simulink model "my_model"  (R2025a)
settings: Solver=FixedStepAuto  StartTime=0.0  StopTime=10.0  RelTol=1e-3
values from neighbouring files (symbols this model uses):
  net = block.UserData    [NN_MPC_SFunction.m]
undefined symbols (not defined in the file or in its folder): getString, message
libraries: dlconvfclib x3, dlactivationlib x2
settings Model: Creator=thapl  LastModifiedBy=thapl
settings OptimizationCC: DefaultParameterBehavior=Inlined  EnhancedBackFolding=on  PassReuseOutputArgsAs=Individual arguments  ZeroExternalMemoryAtStartup=off  ZeroInternalMemoryAtStartup=off  OptimizeBlockOrder=speed  DifferentSizesBufferReuse=on  OptimizationCustomize=off  EfficientTunableParamExpr=on
settings DebuggingCC: ParameterTunabilityLossMsg=error
settings SFSimCC: MATLABDynamicMemAlloc=off
settings RTWCC: SystemTargetFile=ert.tlc  TemplateMakefile=ert_default_tmf  Description=Embedded Coder
settings CodeAppCC: ForceParamTrailComments=on  IgnoreCustomStorageClasses=off  OperatorAnnotations=on  SimulinkDataObjDesc=on  SFDataObjDesc=on  InsertBlockDesc=on
settings ERTTargetCC: ExtModeTransport=0.0  ExtModeStaticAlloc=off  ExtModeMexFile=ext_comm  ExtModeIntrfLevel=Level1  ERTCustomFileTemplate=example_file_process.tlc  TargetLangStandard=C99 (ISO)  GenerateSampleERTMain=on

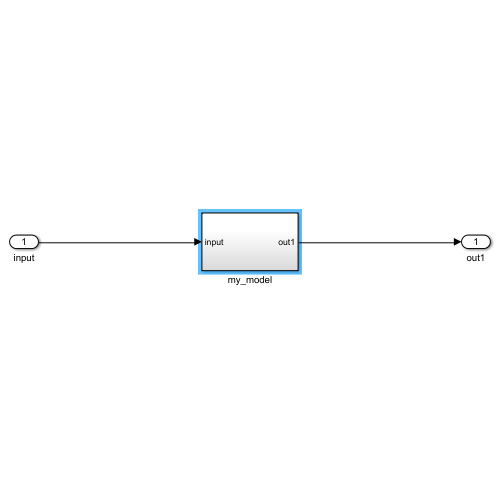
[thumbnail: Simulink's stored preview of the top-level diagram]
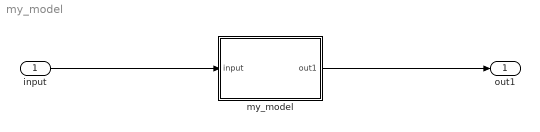
== system my_model ==
  input : Inport  PortDimensions=[20]
  my_model : Subsystem
  out1 : Outport
  wires:
  input/1 -> my_model/1(input)
  my_model/1(out1) -> out1/1

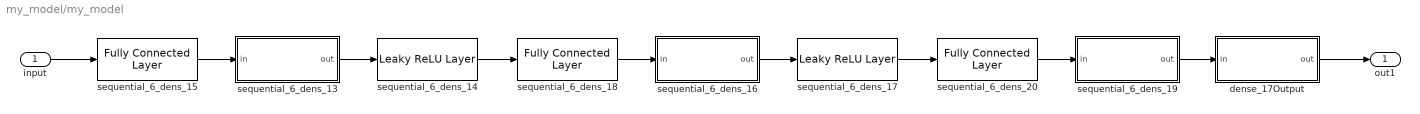
== system my_model/my_model ==
  input : Inport  PortDimensions=[20]
  dense_17Output : Subsystem
  sequential_6_dens_13 : Subsystem
  sequential_6_dens_14 : dlactivationlib/Leaky ReLU Layer  Scale=net.Layers(4).Scale  OutMin=[]  OutMax=[]  ScaleDataTypeStr=Inherit: Inherit via back propagation  ScaleMin=[]  ScaleMax=[]  InternalRndMeth=Floor  InternalSaturateOnIntegerOverflow=off  SampleTime=-1
  sequential_6_dens_15 : dlconvfclib/Fully Connected Layer  Layer=net.Layers(2)  OutMin=[]  OutMax=[]  WeightsDataTypeStr=Inherit: Inherit via back propagation  WeightsMin=[]  WeightsMax=[]  BiasDataTypeStr=Inherit: Inherit via back propagation  BiasMin=[]  BiasMax=[]  AccumMin=[]  AccumMax=[]  InternalRndMeth=Floor  InternalSaturateOnIntegerOverflow=off  SampleTime=-1
      settings: DataFormat=C
  sequential_6_dens_16 : Subsystem
  sequential_6_dens_17 : dlactivationlib/Leaky ReLU Layer  Scale=net.Layers(7).Scale  OutMin=[]  OutMax=[]  ScaleDataTypeStr=Inherit: Inherit via back propagation  ScaleMin=[]  ScaleMax=[]  InternalRndMeth=Floor  InternalSaturateOnIntegerOverflow=off  SampleTime=-1
  sequential_6_dens_18 : dlconvfclib/Fully Connected Layer  Layer=net.Layers(5)  OutMin=[]  OutMax=[]  WeightsDataTypeStr=Inherit: Inherit via back propagation  WeightsMin=[]  WeightsMax=[]  BiasDataTypeStr=Inherit: Inherit via back propagation  BiasMin=[]  BiasMax=[]  AccumMin=[]  AccumMax=[]  InternalRndMeth=Floor  InternalSaturateOnIntegerOverflow=off  SampleTime=-1
      settings: DataFormat=C
  sequential_6_dens_19 : Subsystem
  sequential_6_dens_20 : dlconvfclib/Fully Connected Layer  Layer=net.Layers(8)  OutMin=[]  OutMax=[]  WeightsDataTypeStr=Inherit: Inherit via back propagation  WeightsMin=[]  WeightsMax=[]  BiasDataTypeStr=Inherit: Inherit via back propagation  BiasMin=[]  BiasMax=[]  AccumMin=[]  AccumMax=[]  InternalRndMeth=Floor  InternalSaturateOnIntegerOverflow=off  SampleTime=-1
      settings: DataFormat=C
  out1 : Outport
  wires:
  sequential_6_dens_14/1 -> sequential_6_dens_18/1
  sequential_6_dens_20/1 -> sequential_6_dens_19/1(in)
  sequential_6_dens_17/1 -> sequential_6_dens_20/1
  sequential_6_dens_16/1(out) -> sequential_6_dens_17/1
  sequential_6_dens_18/1 -> sequential_6_dens_16/1(in)
  input/1 -> sequential_6_dens_15/1
  sequential_6_dens_15/1 -> sequential_6_dens_13/1(in)
  dense_17Output/1(out) -> out1/1
  sequential_6_dens_13/1(out) -> sequential_6_dens_14/1
  sequential_6_dens_19/1(out) -> dense_17Output/1(in)

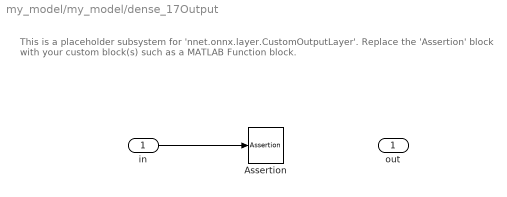
== system my_model/my_model/dense_17Output ==
  note: This is a placeholder subsystem for 'nnet.onnx.layer.CustomOutputLayer'. Replace the 'Assertion' block with your custom block(s) such as a MATLAB Function block.
  in : Inport
  Assertion : Assertion  AssertionFailFcn=disp(getString(message('nnet_layerblocks:deeplayerlib:placeholderSubsystemAssertion', 'nnet.onnx.layer.CustomOutputLayer')))
  out : Outport
  wires:
  in/1 -> Assertion/1

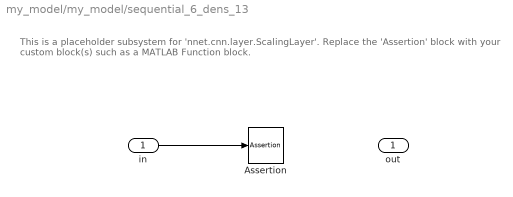
== system my_model/my_model/sequential_6_dens_13 ==
  note: This is a placeholder subsystem for 'nnet.cnn.layer.ScalingLayer'. Replace the 'Assertion' block with your custom block(s) such as a MATLAB Function block.
  in : Inport
  Assertion : Assertion  AssertionFailFcn=disp(getString(message('nnet_layerblocks:deeplayerlib:placeholderSubsystemAssertion', 'nnet.cnn.layer.ScalingLayer')))
  out : Outport
  wires:
  in/1 -> Assertion/1

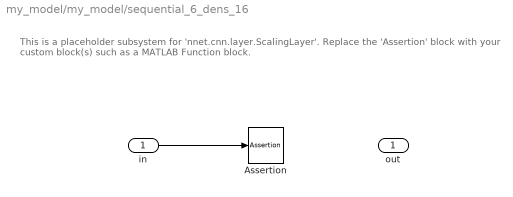
== system my_model/my_model/sequential_6_dens_16 ==
  note: This is a placeholder subsystem for 'nnet.cnn.layer.ScalingLayer'. Replace the 'Assertion' block with your custom block(s) such as a MATLAB Function block.
  in : Inport
  Assertion : Assertion  AssertionFailFcn=disp(getString(message('nnet_layerblocks:deeplayerlib:placeholderSubsystemAssertion', 'nnet.cnn.layer.ScalingLayer')))
  out : Outport
  wires:
  in/1 -> Assertion/1

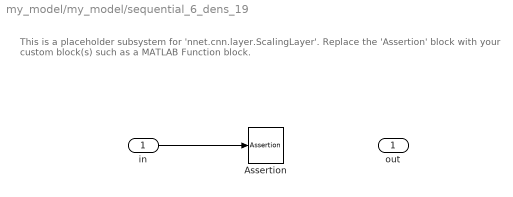
== system my_model/my_model/sequential_6_dens_19 ==
  note: This is a placeholder subsystem for 'nnet.cnn.layer.ScalingLayer'. Replace the 'Assertion' block with your custom block(s) such as a MATLAB Function block.
  in : Inport
  Assertion : Assertion  AssertionFailFcn=disp(getString(message('nnet_layerblocks:deeplayerlib:placeholderSubsystemAssertion', 'nnet.cnn.layer.ScalingLayer')))
  out : Outport
  wires:
  in/1 -> Assertion/1
